simulink model "etc_controller"  (R2022b)
settings: Solver=FixedStepDiscrete  StartTime=0.0  StopTime=10  FixedStep=.01  RelTol=1e-3  EnableMultiTasking=on
PreLoadFcn:
  | % Load Parameters
  | etc_PI_data;
undefined symbols (not defined in the file): Ki, Kp, Ts
Description:
  | This is my help
settings Model: ParamWorkspaceSource=ReferencedWorkspace  Creator=nicholas  LastModifiedBy=bensweet
settings SolverCC: AlgebraicLoopSolver=TrustRegion
settings DataIOCC: LimitDataPoints=on  LoadExternalInput=on  SaveFormat=Array  ReturnWorkspaceOutputs=off  SignalLoggingName=sigsOut
settings OptimizationCC: DefaultParameterBehavior=Inlined  ExpressionDepthLimit=2147483647  InitFltsAndDblsToZero=on  LifeSpan=inf
settings DebuggingCC: UnconnectedInputMsg=warning  UnconnectedOutputMsg=warning  UnconnectedLineMsg=warning  PregeneratedLibrarySubsystemCodeDiagnostic=none  SFMachineParentedDataDiag=warning
settings HardwareCC: ProdBitPerPointer=32  ProdBitPerSizeT=32  ProdBitPerPtrDiffT=32  ProdLargestAtomicFloat=None  ProdIntDivRoundTo=Undefined  ProdEndianess=Unspecified  ProdWordSize=32  ProdHWDeviceType=32-bit Generic  TargetIntDivRoundTo=Zero  TargetEndianess=BigEndian  TargetHWDeviceType=Motorola PowerPC
settings ModelReferenceCC: EnableRefExpFcnMdlSchedulingChecks=on  PropagateSignalLabelsOutOfModel=off
settings SFSimCC: SimUseLocalCustomCode=off
settings RTWCC: RTWUseLocalCustomCode=off  DLArmComputeVersion=19.05
settings CodeAppCC: StateflowObjectComments=on
settings GRTTargetCC: TargetFcnLib=ansi_tfl_tmw.mat  TargetLangStandard=C89/C90 (ANSI)  CombineOutputUpdateFcns=off  GRTInterface=on
settings ConfigComp: CovMetricSettings=dw  CovSaveCumulativeToWorkspaceVar=on  CovSaveSingleToWorkspaceVar=on  CovExternalEMLEnable=off  CovSFcnEnable=off

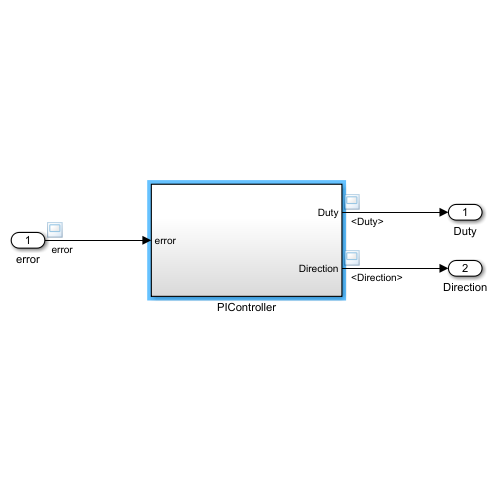
[thumbnail: Simulink's stored preview of the top-level diagram]
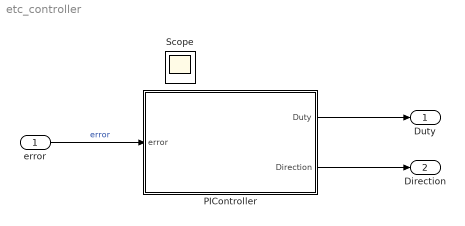
== system etc_controller ==
  error : Inport
  PIController : Subsystem
  Duty : Outport  VectorParamsAs1DForOutWhenUnconnected=off
  Direction : Outport  Port=2  VectorParamsAs1DForOutWhenUnconnected=off
  Scope : Scope
  wires:
  PIController/1(Duty) -> Duty/1
  PIController/2(Direction) -> Direction/1
  error/1 -> PIController/1(error)  "error"

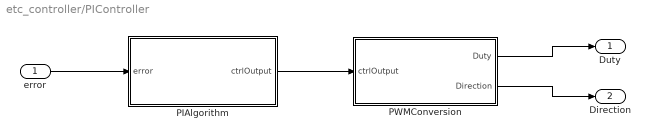
== system etc_controller/PIController ==
  error : Inport  SampleTime=Ts
  PIAlgorithm : Subsystem
  PWMConversion : Subsystem
  Duty : Outport  VectorParamsAs1DForOutWhenUnconnected=off
  Direction : Outport  Port=2  VectorParamsAs1DForOutWhenUnconnected=off
  wires:
  error/1 -> PIAlgorithm/1(error)
  PWMConversion/1(Duty) -> Duty/1
  PWMConversion/2(Direction) -> Direction/1
  PIAlgorithm/1(ctrlOutput) -> PWMConversion/1(ctrlOutput)

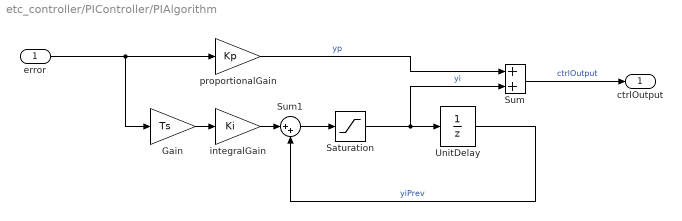
== system etc_controller/PIController/PIAlgorithm ==
  error : Inport  SampleTime=Ts
      settings: AttributesFormatString=Sample time = %<SampleTime>
  Gain : Gain  Gain=Ts  SaturateOnIntegerOverflow=on  OutDataTypeStr=Inherit: Same as input  ParamDataTypeStr=Inherit: Same as input
  Saturation : Saturate  UpperLimit=1  LowerLimit=-1
      settings: AttributesFormatString=Max: %<UpperLimit>\nMin: %<LowerLimit>
  Sum : Sum  InputSameDT=on  SaturateOnIntegerOverflow=on  OutDataTypeStr=Inherit: Same as first input
  Sum1 : Sum  Inputs=|++  InputSameDT=on  SaturateOnIntegerOverflow=on  OutDataTypeStr=Inherit: Same as first input
  UnitDelay : UnitDelay  SampleTime=Ts  HasFrameUpgradeWarning=on
      settings: AttributesFormatString=yi0 = %<X0>\nSample time = %<SampleTime>
  integralGain : Gain  Gain=Ki  SaturateOnIntegerOverflow=on  OutDataTypeStr=Inherit: Same as input  ParamDataTypeStr=Inherit: Same as input
  proportionalGain : Gain  Gain=Kp  SaturateOnIntegerOverflow=on  OutDataTypeStr=Inherit: Same as input  ParamDataTypeStr=Inherit: Same as input
  ctrlOutput : Outport  VectorParamsAs1DForOutWhenUnconnected=off
  wires:
  proportionalGain/1 -> Sum/1  "yp"
  integralGain/1 -> Sum1/1
  Gain/1 -> integralGain/1
  UnitDelay/1 -> Sum1/2  "yiPrev"
  Sum1/1 -> Saturation/1
  Saturation/1 -> UnitDelay/1, Sum/2  "yi"
  error/1 -> proportionalGain/1, Gain/1
  Sum/1 -> ctrlOutput/1  "ctrlOutput"

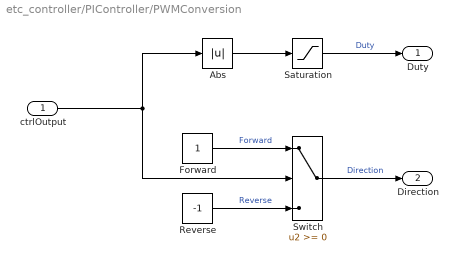
== system etc_controller/PIController/PWMConversion ==
  ctrlOutput : Inport
  Abs : Abs  SaturateOnIntegerOverflow=off
  Forward : Constant  OutDataTypeStr=double
  Reverse : Constant  Value=-1  OutDataTypeStr=double
  Saturation : Saturate  UpperLimit=1  LowerLimit=0
      settings: AttributesFormatString=%<LowerLimit> < duty < %<UpperLimit>
  Switch : Switch  SaturateOnIntegerOverflow=off  InputSameDT=off
      settings: AttributesFormatString=Criteria: %<Criteria>\nThreshold: %<Threshold>
  Duty : Outport  VectorParamsAs1DForOutWhenUnconnected=off
  Direction : Outport  Port=2  VectorParamsAs1DForOutWhenUnconnected=off
  wires:
  Abs/1 -> Saturation/1
  Saturation/1 -> Duty/1  "Duty"
  Switch/1 -> Direction/1  "Direction"
  Reverse/1 -> Switch/3  "Reverse"
  Forward/1 -> Switch/1  "Forward"
  ctrlOutput/1 -> Switch/2, Abs/1
